simulink model "iir_bp_quantization_errors"  (R2018b)
settings: Solver=FixedStepDiscrete  StartTime=0.0  StopTime=0.1  RelTol=1e-3  EnableMultiTasking=on
InitFcn:
  | fs = 48000
undefined symbols (not defined in the file or in its folder): dfilt
libraries: dsparch4 x3, dspsrcs4 x1
settings Model: ExtModeAutoUpdateStatusClock=off  Creator=wolter  LastModifiedBy=wolter
settings DataIOCC: SaveFormat=Array
settings OptimizationCC: ExpressionDepthLimit=2147483647  InitFltsAndDblsToZero=on  LifeSpan=inf
settings DebuggingCC: SaveWithParameterizedLinksMsg=none  SignalResolutionControl=TryResolveAllWithWarning  SolverPrmCheckMsg=warning  MultiTaskDSMMsg=warning  MultiTaskCondExecSysMsg=none  AllowSymbolicDim=off  StateNameClashWarn=warning  SFUnexpectedBacktrackingDiag=warning  SFNoUnconditionalDefaultTransitionDiag=warning  SFExecutionAtInitializationDiag=none
settings HardwareCC: ProdBitPerPointer=32  ProdBitPerSizeT=32  ProdBitPerPtrDiffT=32  ProdLargestAtomicFloat=None  ProdIntDivRoundTo=Undefined  ProdEndianess=Unspecified  ProdWordSize=32  ProdHWDeviceType=32-bit Generic
settings ModelReferenceCC: PropagateSignalLabelsOutOfModel=off
settings SFSimCC: SimUseLocalCustomCode=off
settings RTWCC: RTWUseLocalCustomCode=off
settings CodeAppCC: StateflowObjectComments=on
settings GRTTargetCC: TargetFcnLib=ansi_tfl_tmw.mat  TargetLangStandard=C89/C90 (ANSI)  GeneratePreprocessorConditionals=Disable all  CombineOutputUpdateFcns=off  GRTInterface=on
settings ConfigComp: CovMetricSettings=dw  CovHtmlReporting=on  CovSaveCumulativeToWorkspaceVar=on  CovSaveSingleToWorkspaceVar=on  CovExternalEMLEnable=off

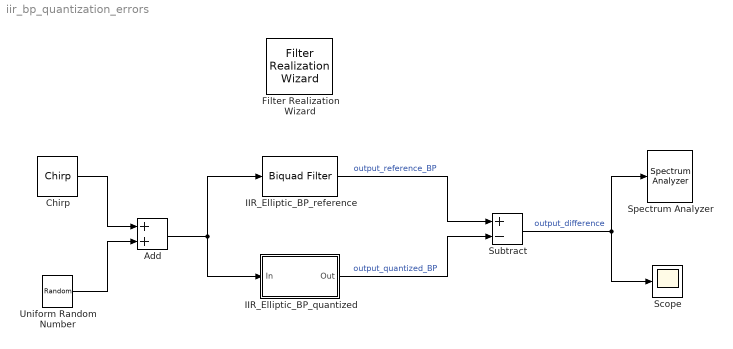
== system iir_bp_quantization_errors ==
  Add : Sum
  Chirp : dspsrcs4/Chirp  sweep=Linear  mode=Unidirectional  f0=1000  f1=20000  t1=0.1  Tsweep=0.1  phase=0  Ts=1/fs  spf=1  datatype=Double  OutputFrames=on
      settings: SourceProductName=DSP System Toolbox
  Filter Realization Wizard : dsparch4/Filter Realization Wizard
      settings: SourceProductName=DSP System Toolbox  SourceProductBaseCode=DS
  IIR_Elliptic_BP_quantized : Subsystem  Tag=BlockMethodSubSystem
  IIR_Elliptic_BP_reference : dsparch4/Biquad Filter  Tag=BlockMethodSubSystem  FilterSource=Dialog parameters  CoeffSource=Specify via dialog  FilterObject=dfilt.df2tsos([1 0.3 0.4],[1 0.1 0.2])  IIRFiltStruct=Direct form II  BiQuadCoeffs=[1 -1.19425971532663 1 1 -0.93026968865773 0.958029078099323;1 0.528447151377372 1 1 0.191934789534485 0.952662991261437;1 -1.38081431779474 1 1 -0.787284236121172 0.913142080510581;1 0.811816164990394 1 1 0.0369568533569792 0.905116377331925;1 1.63742511269465 1 1 -0.225279475008985 0.862272962059629;1 -1.8343474981565 1 1 -0.537781414297456 0.866811928299307;1 -1.13272784244798 1 1 -0.993252493405691 0.988058582903498;1 0.440887112115382 1 1 0.258252858975978 0.986343625511385]  ScaleValues=[0.761322086582269;0.761322086582269;0.704985418970828;0.704985418970828;0.654630520350488;0.654630520350488;0.064744332148743;0.064744332148743;1]  IC=0  ICnum=0  ICden=0  a0Flag=Warning  optimizeScaleValues=on  ScaleValueMode=Specify via input port (g)  InputProcessing=Columns as channels (frame based)  roundingMode=Floor  overflowMode=off  scaleValueFracLength=14  denProdOutputFracLength=30  denAccumFracLength=30  secondMemoryFracLength=15
      settings: SourceProductName=DSP System Toolbox
  Scope : Scope
  Spectrum Analyzer : SpectrumAnalyzer
  Subtract : Sum  Inputs=+-
  Uniform Random Number : UniformRandomNumber  Minimum=-0.5  Maximum=0.5  SampleTime=1/fs
  wires:
  Add/1 -> IIR_Elliptic_BP_reference/1, IIR_Elliptic_BP_quantized/1(In)
  Chirp/1 -> Add/1
  Uniform Random Number/1 -> Add/2
  IIR_Elliptic_BP_reference/1 -> Subtract/1  "output_reference_BP"
  IIR_Elliptic_BP_quantized/1(Out) -> Subtract/2  "output_quantized_BP"
  Subtract/1 -> Scope/1, Spectrum Analyzer/1  "output_difference"

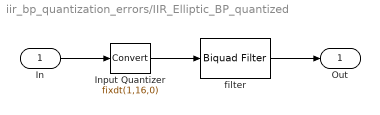
== system iir_bp_quantization_errors/IIR_Elliptic_BP_quantized ==
  In : Inport
  Input Quantizer : DataTypeConversion  OutDataTypeStr=fixdt(1,16,0)  RndMeth=Round  SaturateOnIntegerOverflow=on
  filter : dsparch4/Biquad Filter  FilterSource=Dialog parameters  CoeffSource=Specify via dialog  FilterObject=dfilt.df2tsos([1 0.3 0.4],[1 0.1 0.2])  IIRFiltStruct=Direct form II  BiQuadCoeffs=[1 -1.19425971532663 1 1 -0.93026968865773 0.958029078099323;1 0.528447151377372 1 1 0.191934789534485 0.952662991261437;1 -1.38081431779474 1 1 -0.787284236121172 0.913142080510581;1 0.811816164990394 1 1 0.0369568533569792 0.905116377331925;1 1.63742511269465 1 1 -0.225279475008985 0.862272962059629;1 -1.8343474981565 1 1 -0.537781414297456 0.866811928299307;1 -1.13272784244798 1 1 -0.993252493405691 0.988058582903498;1 0.440887112115382 1 1 0.258252858975978 0.986343625511385]  ScaleValues=[0.761322086582269;0.761322086582269;0.704985418970828;0.704985418970828;0.654630520350488;0.654630520350488;0.064744332148743;0.064744332148743;1]  IC=0  ICnum=0  ICden=0  a0Flag=Warning  optimizeScaleValues=on  ScaleValueMode=Specify via input port (g)  InputProcessing=Columns as channels (frame based)  roundingMode=Convergent  overflowMode=off  stageInputMode=Binary point scaling  stageInputWordLength=16  stageInputFracLength=15  stageOutputMode=Binary point scaling  stageOutputWordLength=16  stageOutputFracLength=15  firstCoeffMode=Binary point scaling  firstCoeffWordLength=8  firstCoeffFracLength=7  scaleValueFracLength=7  prodOutputMode=Binary point scaling  prodOutputWordLength=24  prodOutputFracLength=21  denProdOutputFracLength=21  accumMode=Binary point scaling  accumWordLength=40  accumFracLength=21  denAccumFracLength=21  memoryMode=Binary point scaling  memoryWordLength=16  memoryFracLength=15  secondMemoryFracLength=15  outputMode=Binary point scaling  outputWordLength=16  outputFracLength=11
      settings: SourceProductName=DSP System Toolbox
  Out : Outport
  wires:
  In/1 -> Input Quantizer/1
  Input Quantizer/1 -> filter/1
  filter/1 -> Out/1
